simulink model "ArduinoMain"  (R2013a)
settings: Solver=ode3  SolverMode=SingleTasking  StartTime=0.0  StopTime=inf  RelTol=1e-3
PreLoadFcn:
  | load sensorbus
model workspace (MAT data in the model file):
  hc = 23
  zc = -18
  lc = -59
  hsl = -5
  lsl = -28
  rc = 82
undefined symbols (not defined in the file or in its folder): magnitude, sigbuilder_block
libraries: arduinolib x43, simulink x21
settings Model: SimulationMode=external  ExtModeTrigDuration=2  Creator=sbiagion  LastModifiedBy=user
settings OptimizationCC: OptimizeModelRefInitCode=on  LifeSpan=1
settings DebuggingCC: SolverPrmCheckMsg=none  StrictBusMsg=Warning  SFUnusedDataAndEventsDiag=none
settings HardwareCC: ProdBitPerInt=16  ProdBitPerPointer=8  ProdIntDivRoundTo=Zero  ProdEndianess=LittleEndian  ProdWordSize=8  ProdHWDeviceType=Atmel->AVR
settings RTWCC: SystemTargetFile=realtime.tlc  GenerateMakefile=off  TemplateMakefile=realtime.tmf  Description=Run on Target Hardware  RTWVerbose=off  ProcessScript=realtime_make_rtw_hook
settings STFCustomTargetCC: TargetLibSuffix=.a  GenerateSampleERTMain=on  ERTCustomFileBanners=on  SupportNonInlinedSFcns=off  SupportVariableSizeSignals=on  MATLABClassNameForMDSCustomization=Simulink.SoftwareTarget.ERTCustomization  SystemTargetFile=realtime.tlc
settings ERTTargetCC: ParMdlRefBuildCompliant=off  CompOptLevelCompliant=off  ConcurrentExecutionCompliant=off  CombineOutputUpdateFcns=off  ERTFirstTimeCompliant=off  SupportContinuousTime=on  SupportVariableSizeSignals=on  ModelStepFunctionPrototypeControlCompliant=off  CPPClassGenCompliant=off  ExtModeTransport=3  ExtModeMexFile=ext_serial_win32_comm  ExtModeMexArgs=0 15 115200  ERTSrcFileBannerTemplate=realtime_code_template.cgt  ERTHdrFileBannerTemplate=realtime_code_template.cgt  ERTDataSrcFileTemplate=realtime_code_template.cgt  ERTDataHdrFileTemplate=realtime_code_template.cgt  ERTCustomFileTemplate=realtime_file_process.tlc

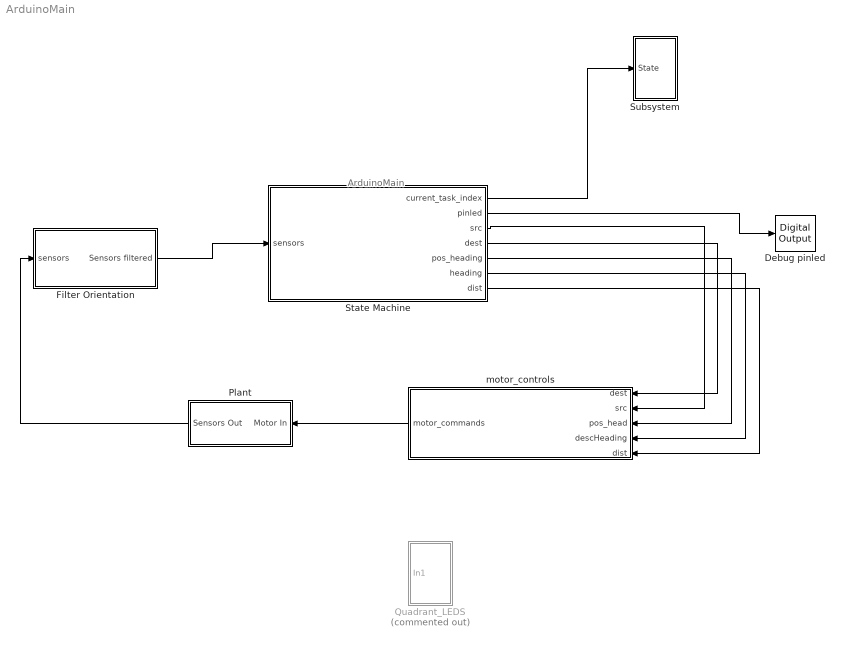
== system ArduinoMain ==
  note: ArduinoMain
  Debug pinled : arduinolib/Digital Output  pinNumber=13
  Filter Orientation : Subsystem
  Plant : Subsystem
  Quadrant_LEDS : Subsystem  Commented=on
  State Machine : Stateflow chart  TreatAsAtomicUnit=on
  Subsystem : Subsystem
  "motor_controls " : Subsystem
  wires:
  State Machine/2(pinled) -> Debug pinled/1
  Plant/1(Sensors Out) -> Filter Orientation/1(sensors)
  Filter Orientation/1(Sensors filtered) -> State Machine/1(sensors)
  "motor_controls "/1("motor_commands ") -> Plant/1(Motor In)
  State Machine/3(src) -> "motor_controls "/2("src ")
  State Machine/4(dest) -> "motor_controls "/1("dest ")
  State Machine/5(pos_heading) -> "motor_controls "/3(pos_head)
  State Machine/6(heading) -> "motor_controls "/4("descHeading ")
  State Machine/7(dist) -> "motor_controls "/5(dist)
  State Machine/1(current_task_index) -> Subsystem/1("State ")

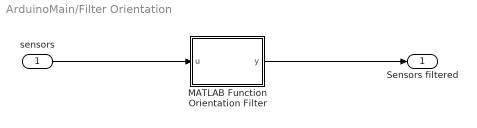
== system ArduinoMain/Filter Orientation ==
  sensors : Inport
  MATLAB Function Orientation Filter : MATLAB Function  TreatAsAtomicUnit=on
  Sensors filtered : Outport
  wires:
  sensors/1 -> MATLAB Function Orientation Filter/1(u)
  MATLAB Function Orientation Filter/1(y) -> Sensors filtered/1

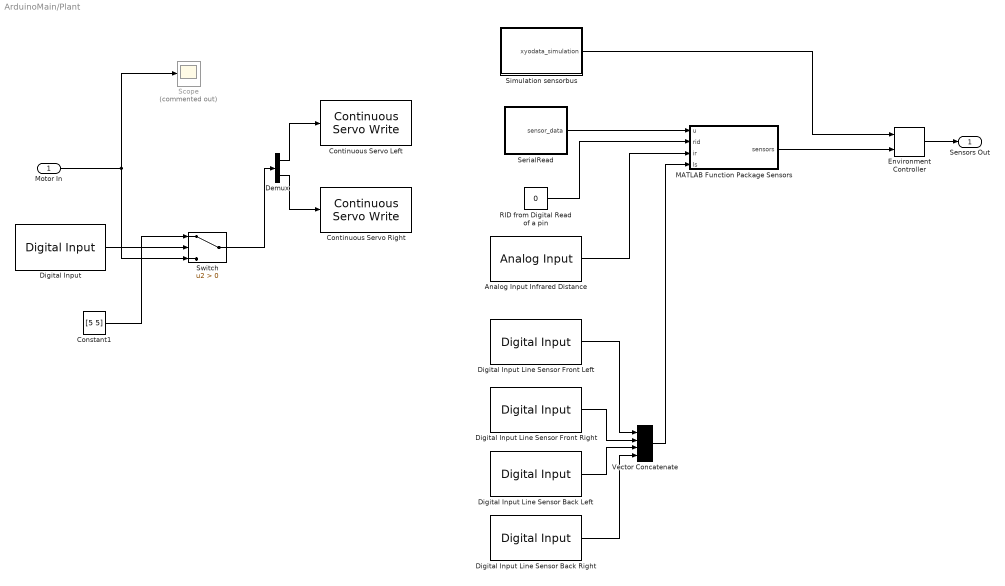
== system ArduinoMain/Plant ==
  Motor In : Inport
  Analog Input Infrared Distance : arduinolib/Analog Input  pinNumber=0  sampleTime=0.01
  Constant1 : Constant  Value=[5 5]
  Continuous Servo Left : arduinolib/Continuous Servo Write  pinNumber=50
  Continuous Servo Right : arduinolib/Continuous Servo Write  pinNumber=51
  Demux : Demux  Outputs=2
  Digital Input : arduinolib/Digital Input  pinNumber=8  sampleTime=1
  Digital Input Line Sensor Back Left : arduinolib/Digital Input  pinNumber=10  sampleTime=0.001
  Digital Input Line Sensor Back Right : arduinolib/Digital Input  pinNumber=11  sampleTime=0.001
  Digital Input Line Sensor Front Left : arduinolib/Digital Input  pinNumber=20  sampleTime=0.001
  Digital Input Line Sensor Front Right : arduinolib/Digital Input  pinNumber=9  sampleTime=0.001
  Environment Controller : simulink/Signal Routing/Environment Controller
  MATLAB Function Package Sensors : MATLAB Function  TreatAsAtomicUnit=on
  RID from Digital Read of a pin : Constant  Value=0  OutDataTypeStr=single  SampleTime=0.001
  Scope : Scope  Commented=on
      settings: ShowLegends=on  YMin=0  YMax=90
  SerialRead : Subsystem
  Simulation sensorbus : Subsystem
  Switch : Switch  Criteria=u2 > Threshold
  Vector Concatenate : Concatenate  NumInputs=4  Mode=Multidimensional array  ConcatenateDimension=2
  Sensors Out : Outport
  wires:
  Demux/2 -> Continuous Servo Right/1
  Demux/1 -> Continuous Servo Left/1
  Motor In/1 -> Scope/1, Switch/3
  Environment Controller/1 -> Sensors Out/1
  Simulation sensorbus/1(xyodata_simulation) -> Environment Controller/1
  Digital Input Line Sensor Front Left/1 -> Vector Concatenate/1
  Digital Input Line Sensor Front Right/1 -> Vector Concatenate/2
  Digital Input Line Sensor Back Left/1 -> Vector Concatenate/3
  Digital Input Line Sensor Back Right/1 -> Vector Concatenate/4
  RID from Digital Read of a pin/1 -> MATLAB Function Package Sensors/2(rid)
  Analog Input Infrared Distance/1 -> MATLAB Function Package Sensors/3(ir)
  Vector Concatenate/1 -> MATLAB Function Package Sensors/4(ls)
  MATLAB Function Package Sensors/1(sensors) -> Environment Controller/2
  SerialRead/1(sensor_data) -> MATLAB Function Package Sensors/1(u)
  Switch/1 -> Demux/1
  Digital Input/1 -> Switch/2
  Constant1/1 -> Switch/1

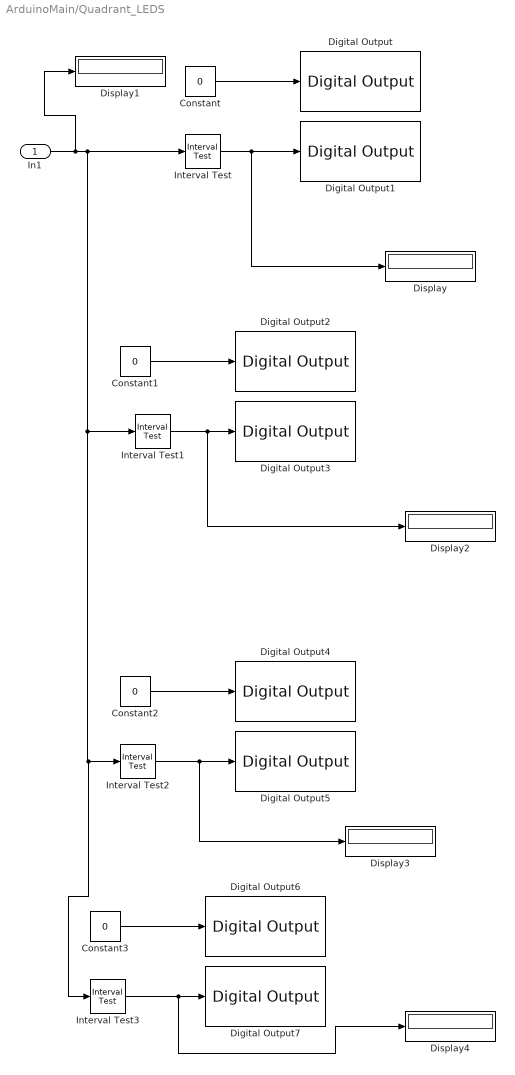
== system ArduinoMain/Quadrant_LEDS ==
  In1 : Inport
  Constant{,1..3} (4 alike) : Constant  Value=0
  Digital Output : arduinolib/Digital Output  pinNumber=23
  Digital Output1 : arduinolib/Digital Output  pinNumber=22
  Digital Output2 : arduinolib/Digital Output  pinNumber=25
  Digital Output3 : arduinolib/Digital Output  pinNumber=24
  Digital Output4 : arduinolib/Digital Output  pinNumber=31
  Digital Output5 : arduinolib/Digital Output  pinNumber=30
  Digital Output6 : arduinolib/Digital Output  pinNumber=29
  Digital Output7 : arduinolib/Digital Output  pinNumber=28
  Display{,1..4} (5 alike) : Display
  Interval Test : simulink/Logic and Bit Operations/Interval Test  IntervalClosedRight=off  uplimit=90  IntervalClosedLeft=on  lowlimit=0  OutDataTypeStr=boolean
  Interval Test1 : simulink/Logic and Bit Operations/Interval Test  IntervalClosedRight=on  uplimit=180  IntervalClosedLeft=on  lowlimit=90  OutDataTypeStr=boolean
  Interval Test2 : simulink/Logic and Bit Operations/Interval Test  IntervalClosedRight=off  uplimit=0  IntervalClosedLeft=on  lowlimit=-90  OutDataTypeStr=boolean
  Interval Test3 : simulink/Logic and Bit Operations/Interval Test  IntervalClosedRight=on  uplimit=-90  IntervalClosedLeft=on  lowlimit=-180  OutDataTypeStr=boolean
  wires:
  Constant/1 -> Digital Output/1
  Interval Test1/1 -> Display2/1, Digital Output3/1
  Constant1/1 -> Digital Output2/1
  Interval Test2/1 -> Display3/1, Digital Output5/1
  Constant2/1 -> Digital Output4/1
  Interval Test/1 -> Display/1, Digital Output1/1
  Interval Test3/1 -> Display4/1, Digital Output7/1
  Constant3/1 -> Digital Output6/1
  In1/1 -> Display1/1, Interval Test/1, Interval Test3/1, Interval Test2/1, Interval Test1/1

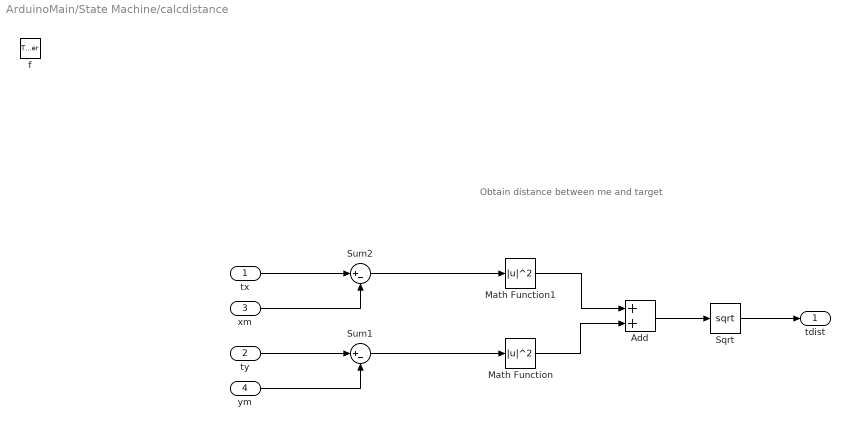
== system ArduinoMain/State Machine/calcdistance ==
  note: Obtain distance between me and target
  tx : Inport  OutDataTypeStr=single  PortDimensions=1
  ty : Inport  Port=2  OutDataTypeStr=single  PortDimensions=1
  xm : Inport  Port=3  OutDataTypeStr=single  PortDimensions=1
  ym : Inport  Port=4  OutDataTypeStr=single  PortDimensions=1
  f : TriggerPort  TriggerType=function-call
      settings: CopyFcn=Stateflow.SLINSF.SimulinkMan.removeBlockPreDeleteFcn  PreDeleteFcn=Stateflow.SLINSF.SimulinkMan.unsafePredeleteFcn
  Add : Sum
  Math Function : Math  Operator=magnitude^2  SaturateOnIntegerOverflow=on
  Math Function1 : Math  Operator=magnitude^2  SaturateOnIntegerOverflow=on
  Sqrt : Sqrt  SaturateOnIntegerOverflow=on
  Sum1 : Sum  Inputs=|+-
  Sum2 : Sum  Inputs=|+-
  tdist : Outport
  wires:
  ty/1 -> Sum1/1
  ym/1 -> Sum1/2
  tx/1 -> Sum2/1
  xm/1 -> Sum2/2
  Sum1/1 -> Math Function/1
  Sum2/1 -> Math Function1/1
  Add/1 -> Sqrt/1
  Math Function1/1 -> Add/1
  Math Function/1 -> Add/2
  Sqrt/1 -> tdist/1

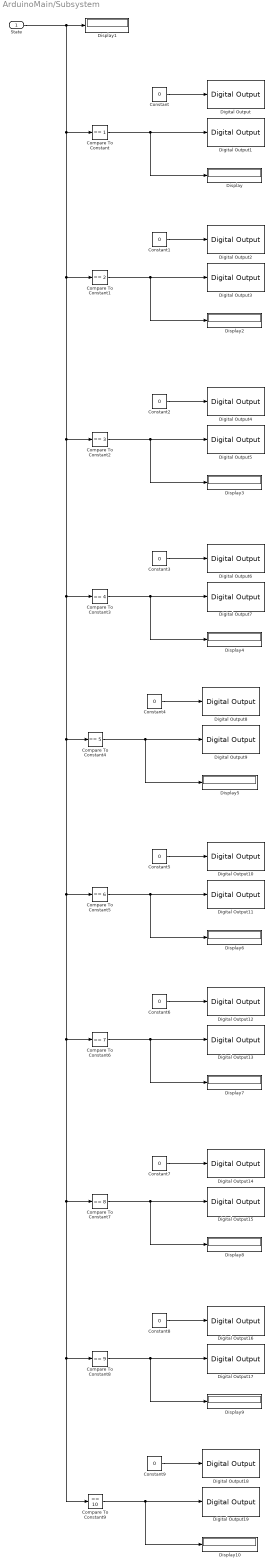
== system ArduinoMain/Subsystem ==
  "State " : Inport
  Compare To Constant : simulink/Logic and Bit Operations/Compare To Constant  relop===  const=1  OutDataTypeStr=boolean
  Compare To Constant1 : simulink/Logic and Bit Operations/Compare To Constant  relop===  const=2  OutDataTypeStr=boolean
  Compare To Constant2 : simulink/Logic and Bit Operations/Compare To Constant  relop===  const=3  OutDataTypeStr=boolean
  Compare To Constant3 : simulink/Logic and Bit Operations/Compare To Constant  relop===  const=4  OutDataTypeStr=boolean
  Compare To Constant4 : simulink/Logic and Bit Operations/Compare To Constant  relop===  const=5  OutDataTypeStr=boolean
  Compare To Constant5 : simulink/Logic and Bit Operations/Compare To Constant  relop===  const=6  OutDataTypeStr=boolean
  Compare To Constant6 : simulink/Logic and Bit Operations/Compare To Constant  relop===  const=7  OutDataTypeStr=boolean
  Compare To Constant7 : simulink/Logic and Bit Operations/Compare To Constant  relop===  const=8  OutDataTypeStr=boolean
  Compare To Constant8 : simulink/Logic and Bit Operations/Compare To Constant  relop===  const=9  OutDataTypeStr=boolean
  Compare To Constant9 : simulink/Logic and Bit Operations/Compare To Constant  relop===  const=10  OutDataTypeStr=boolean
  Constant{,1..9} (10 alike) : Constant  Value=0
  Digital Output : arduinolib/Digital Output  pinNumber=23
  Digital Output1 : arduinolib/Digital Output  pinNumber=22
  Digital Output10 : arduinolib/Digital Output  pinNumber=33
  Digital Output11 : arduinolib/Digital Output  pinNumber=32
  Digital Output12 : arduinolib/Digital Output  pinNumber=35
  Digital Output13 : arduinolib/Digital Output  pinNumber=34
  Digital Output14 : arduinolib/Digital Output  pinNumber=37
  Digital Output15 : arduinolib/Digital Output  pinNumber=36
  Digital Output16 : arduinolib/Digital Output  pinNumber=39
  Digital Output17 : arduinolib/Digital Output  pinNumber=38
  Digital Output18 : arduinolib/Digital Output  pinNumber=41
  Digital Output19 : arduinolib/Digital Output  pinNumber=40
  Digital Output2 : arduinolib/Digital Output  pinNumber=25
  Digital Output3 : arduinolib/Digital Output  pinNumber=24
  Digital Output4 : arduinolib/Digital Output  pinNumber=27
  Digital Output5 : arduinolib/Digital Output  pinNumber=26
  Digital Output6 : arduinolib/Digital Output  pinNumber=29
  Digital Output7 : arduinolib/Digital Output  pinNumber=28
  Digital Output8 : arduinolib/Digital Output  pinNumber=31
  Digital Output9 : arduinolib/Digital Output  pinNumber=30
  Display{,1..10} (11 alike) : Display
  wires:
  Constant/1 -> Digital Output/1
  Compare To Constant/1 -> Display/1, Digital Output1/1
  Constant1/1 -> Digital Output2/1
  Compare To Constant1/1 -> Display2/1, Digital Output3/1
  Constant2/1 -> Digital Output4/1
  Compare To Constant2/1 -> Display3/1, Digital Output5/1
  Constant3/1 -> Digital Output6/1
  Compare To Constant3/1 -> Display4/1, Digital Output7/1
  Constant4/1 -> Digital Output8/1
  Compare To Constant4/1 -> Display5/1, Digital Output9/1
  Constant5/1 -> Digital Output10/1
  Compare To Constant5/1 -> Display6/1, Digital Output11/1
  Constant6/1 -> Digital Output12/1
  Compare To Constant6/1 -> Display7/1, Digital Output13/1
  Constant7/1 -> Digital Output14/1
  Compare To Constant7/1 -> Display8/1, Digital Output15/1
  "State "/1 -> Compare To Constant9/1, Compare To Constant8/1, Compare To Constant7/1, Compare To Constant6/1, Compare To Constant5/1, Compare To Constant4/1, Compare To Constant3/1, Compare To Constant2/1, Compare To Constant1/1, Compare To Constant/1, Display1/1
  Constant8/1 -> Digital Output16/1
  Compare To Constant8/1 -> Display9/1, Digital Output17/1
  Constant9/1 -> Digital Output18/1
  Compare To Constant9/1 -> Display10/1, Digital Output19/1

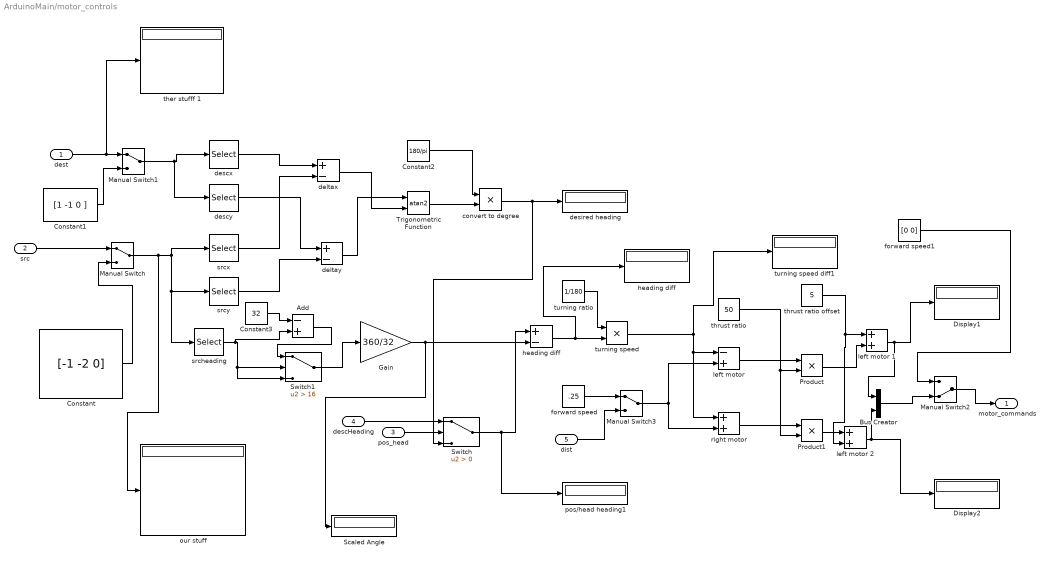
== system ArduinoMain/motor_controls  ==
  "dest " : Inport
  "src " : Inport  Port=2
  pos_head : Inport  Port=3  OutDataTypeStr=boolean
  "descHeading " : Inport  Port=4
  dist : Inport  Port=5
  Add : Sum  Inputs=-+
  Bus Creator : BusCreator  Inputs=2
  Constant : Constant  Value=[-1 -2 0]
  Constant1 : Constant  Value=[1 -1 0 ]
  Constant2 : Constant  Value=180/pi
  Constant3 : Constant  Value=32
  Display1 : Display
  Display2 : Display
  Gain : Gain  Gain=360/32
  Manual Switch : ManualSwitch
  Manual Switch1 : ManualSwitch
  Manual Switch2 : ManualSwitch  CurrentSetting=0
  Manual Switch3 : ManualSwitch
  Product : Product
  Product1 : Product
  Scaled Angle : Display
  Switch : Switch  Criteria=u2 > Threshold
  Switch1 : Switch  Criteria=u2 > Threshold  Threshold=16
  Trigonometric Function : Trigonometry  Operator=atan2
  "convert to degree " : Product
  deltax : Sum  Inputs=+-
  deltay : Sum  Inputs=+-
  "descx " : Selector  InputPortWidth=3  IndexOptions=Index vector (dialog)  Indices=1  OutputSizes=1
  "descy " : Selector  InputPortWidth=3  IndexOptions=Index vector (dialog)  Indices=2  OutputSizes=1
  "desired heading " : Display
  forward speed : Constant  Value=.25
  forward speed1 : Constant  Value=[0 0]
  heading diff : Display
  "heading diff " : Sum  Inputs=+-
  "left motor " : Sum  Inputs=-+
  left motor 1 : Sum
  left motor 2 : Sum
  "our stuff " : Display
  pos/head heading1 : Display
  "right motor " : Sum
  "srcheading " : Selector  InputPortWidth=3  IndexOptions=Index vector (dialog)  Indices=3  OutputSizes=1
  "srcx " : Selector  InputPortWidth=3  IndexOptions=Index vector (dialog)  Indices=1  OutputSizes=1
  "srcy " : Selector  InputPortWidth=3  IndexOptions=Index vector (dialog)  Indices=2  OutputSizes=1
  ther stufff 1 : Display
  "thrust ratio " : Constant  Value=50
  thrust ratio offset : Constant  Value=5
  turning ratio : Constant  Value=1/180
  turning speed : Product
  turning speed diff1 : Display
  "motor_commands " : Outport
  wires:
  "descx "/1 -> deltax/1
  "srcx "/1 -> deltax/2
  "descy "/1 -> deltay/1
  "srcy "/1 -> deltay/2
  deltax/1 -> Trigonometric Function/2
  deltay/1 -> Trigonometric Function/1
  Trigonometric Function/1 -> "convert to degree "/2
  "convert to degree "/1 -> Switch/3, "desired heading "/1
  Constant2/1 -> "convert to degree "/1
  "heading diff "/1 -> turning speed/2, heading diff/1
  turning ratio/1 -> turning speed/1
  turning speed/1 -> turning speed diff1/1, "right motor "/1, "left motor "/1
  "left motor "/1 -> Product/1
  "right motor "/1 -> Product1/1
  "thrust ratio "/1 -> Product1/2, Product/2
  pos_head/1 -> Switch/2
  Switch/1 -> pos/head heading1/1, "heading diff "/1
  Product/1 -> left motor 1/2
  left motor 1/1 -> Bus Creator/1, Display1/1
  thrust ratio offset/1 -> left motor 2/2, left motor 1/1
  Product1/1 -> left motor 2/1
  left motor 2/1 -> Display2/1, Bus Creator/2
  "dest "/1 -> ther stufff 1/1, Manual Switch1/1
  Manual Switch1/1 -> "descy "/1, "descx "/1
  "src "/1 -> Manual Switch/1
  Manual Switch/1 -> "our stuff "/1, "srcx "/1, "srcheading "/1, "srcy "/1
  Constant/1 -> Manual Switch/2
  Constant1/1 -> Manual Switch1/2
  Bus Creator/1 -> Manual Switch2/2
  Manual Switch2/1 -> "motor_commands "/1
  forward speed1/1 -> Manual Switch2/1
  "descHeading "/1 -> Switch/1
  forward speed/1 -> Manual Switch3/1
  Manual Switch3/1 -> "left motor "/2, "right motor "/2
  dist/1 -> Manual Switch3/2
  "srcheading "/1 -> Add/2, Switch1/3, Switch1/2
  Switch1/1 -> Gain/1
  Add/1 -> Switch1/1
  Constant3/1 -> Add/1
  Gain/1 -> Scaled Angle/1, "heading diff "/2

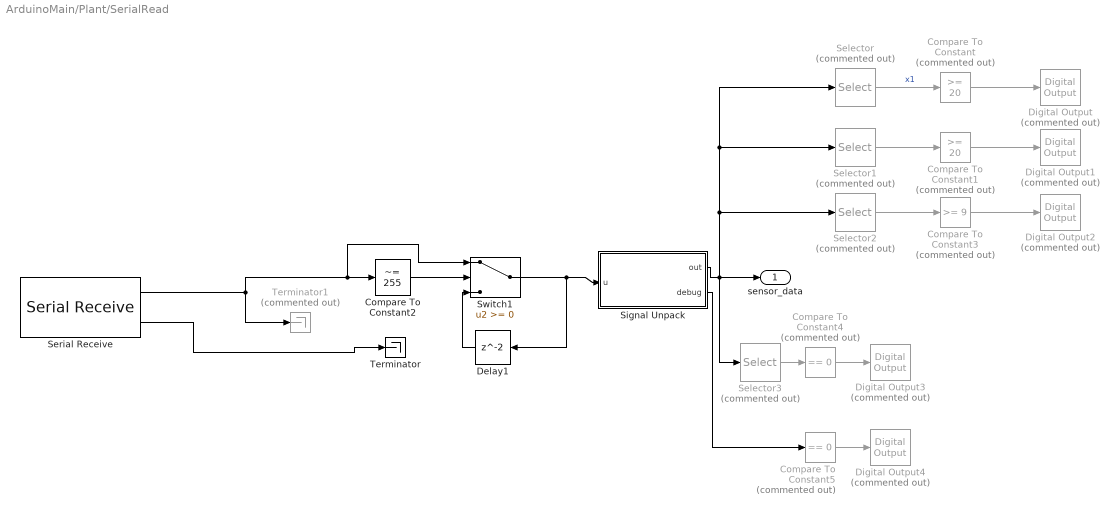
== system ArduinoMain/Plant/SerialRead ==
  Compare To Constant : simulink/Logic and Bit Operations/Compare To Constant  Commented=on  relop=>=  const=20  OutDataTypeStr=boolean
  Compare To Constant1 : simulink/Logic and Bit Operations/Compare To Constant  Commented=on  relop=>=  const=20  OutDataTypeStr=boolean
  Compare To Constant2 : simulink/Logic and Bit Operations/Compare To Constant  relop=~=  const=255  OutDataTypeStr=boolean
  Compare To Constant3 : simulink/Logic and Bit Operations/Compare To Constant  Commented=on  relop=>=  const=9  OutDataTypeStr=boolean
  Compare To Constant4 : simulink/Logic and Bit Operations/Compare To Constant  Commented=on  relop===  const=0  OutDataTypeStr=boolean
  Compare To Constant5 : simulink/Logic and Bit Operations/Compare To Constant  Commented=on  relop===  const=0  OutDataTypeStr=boolean
  Delay1 : Delay
  Digital Output : arduinolib/Digital Output  Commented=on  pinNumber=12
  Digital Output1 : arduinolib/Digital Output  Commented=on  pinNumber=11
  Digital Output2 : arduinolib/Digital Output  Commented=on  pinNumber=10
  Digital Output3 : arduinolib/Digital Output  Commented=on  pinNumber=9
  Digital Output4 : arduinolib/Digital Output  Commented=on  pinNumber=9
  Selector : Selector  Commented=on  InputPortWidth=7  IndexOptions=Index vector (dialog)  Indices=1  OutputSizes=1
  Selector1 : Selector  Commented=on  InputPortWidth=7  IndexOptions=Index vector (dialog)  Indices=2  OutputSizes=1
  Selector2 : Selector  Commented=on  InputPortWidth=7  IndexOptions=Index vector (dialog)  Indices=3  OutputSizes=1
  Selector3 : Selector  Commented=on  InputPortWidth=7  IndexOptions=Index vector (dialog)  Indices=7  OutputSizes=1
  Serial Receive : arduinolib/Serial Receive  portNumber=1  showOutStatus=on  sampleTime=0.001
  Signal Unpack : MATLAB Function  TreatAsAtomicUnit=on
  Switch1 : Switch
  Terminator : Terminator
  Terminator1 : Terminator  Commented=on
  sensor_data : Outport
  wires:
  Switch1/1 -> Delay1/1, Signal Unpack/1(u)
  Compare To Constant2/1 -> Switch1/2
  Serial Receive/2 -> Terminator/1
  Delay1/1 -> Switch1/3
  Serial Receive/1 -> Terminator1/1, Switch1/1, Compare To Constant2/1
  Selector/1 -> Compare To Constant/1  "x1"
  Compare To Constant/1 -> Digital Output/1
  Compare To Constant1/1 -> Digital Output1/1
  Selector1/1 -> Compare To Constant1/1
  Selector2/1 -> Compare To Constant3/1
  Compare To Constant3/1 -> Digital Output2/1
  Selector3/1 -> Compare To Constant4/1
  Signal Unpack/1(out) -> Selector3/1, Selector/1, Selector1/1, Selector2/1, sensor_data/1
  Compare To Constant4/1 -> Digital Output3/1
  Signal Unpack/2(debug) -> Compare To Constant5/1
  Compare To Constant5/1 -> Digital Output4/1

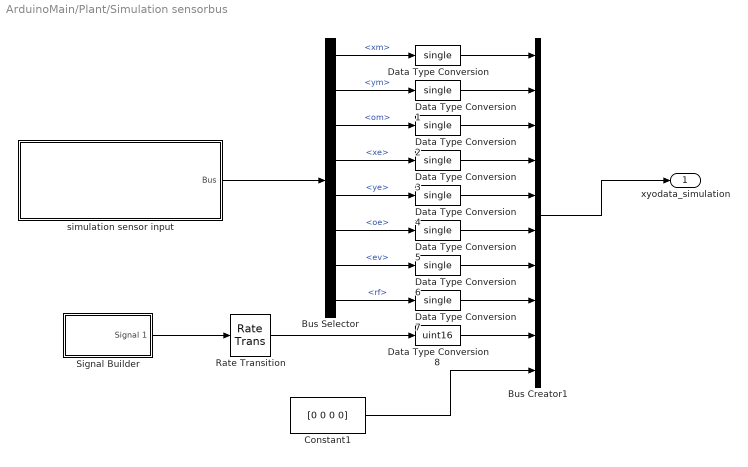
== system ArduinoMain/Plant/Simulation sensorbus ==
  Bus Creator1 : BusCreator  Inputs=10  OutDataTypeStr=Bus: sensorbus  NonVirtualBus=on
  Bus Selector : BusSelector  OutputSignals=xm,ym,om,xe,ye,oe,ev,rf
  Constant1 : Constant  Value=[0 0 0 0]  OutDataTypeStr=boolean
  Data Type Conversion{,1..7} (8 alike) : DataTypeConversion  OutDataTypeStr=single
  Data Type Conversion8 : DataTypeConversion  OutDataTypeStr=uint16
  Rate Transition : RateTransition  Integrity=off
  Signal Builder : Subsystem  Tag=STV Subsys  LoadFcn=sigbuilder_block('load');  StartFcn=sigbuilder_block('start');  StopFcn=sigbuilder_block('stop');  ClipboardFcn=sigbuilder_block('clipboard');  mask(Sigbuilder block){}
      mask help: Simulink:masks:SigbuilderBlock_MD
      mask init:
      | if ~strcmp(get_param(bdroot(gcbh),'SimulationStatus'),'stopped') tuvar = sigbuilder_block('maskInit'); end
      settings: CopyFcn=sigbuilder_block('copy');  DeleteFcn=sigbuilder_block('delete');  ModelCloseFcn=sigbuilder_block('modelClose');  PreSaveFcn=sigbuilder_block('preSave');  PauseFcn=sigbuilder_block('pause');  ContinueFcn=sigbuilder_block('continue');  NameChangeFcn=sigbuilder_block('namechange');  OpenFcn=sigbuilder_block('open',[437.25 199.5 550.5 399.75 ]);  CloseFcn=sigbuilder_block('close');
      mask Display: plot(0, 0, 100, 100,[2, 2, 32, 32, 2], [68, 8, 8, 68, 68],[32, 2], [38, 38], [32, 19, 2],[53, 60, 44], [32, 17, 17, 2],[16, 16, 31, 31]);txt = getActiveGroup(gcbh);text(2, 100, txt,'verticalAlignment', 'top');
  simulation sensor input : Subsystem  Tag=STV Subsys  LoadFcn=sigbuilder_block('load');  StartFcn=sigbuilder_block('start');  StopFcn=sigbuilder_block('stop');  ClipboardFcn=sigbuilder_block('clipboard');  mask(Sigbuilder block){}
      mask help: Simulink:masks:SigbuilderBlock_MD
      mask init:
      | if ~strcmp(get_param(bdroot(gcbh),'SimulationStatus'),'stopped') tuvar = sigbuilder_block('maskInit'); end
      settings: CopyFcn=sigbuilder_block('copy');  DeleteFcn=sigbuilder_block('delete');  ModelCloseFcn=sigbuilder_block('modelClose');  PreSaveFcn=sigbuilder_block('preSave');  PauseFcn=sigbuilder_block('pause');  ContinueFcn=sigbuilder_block('continue');  NameChangeFcn=sigbuilder_block('namechange');  OpenFcn=sigbuilder_block('open',[6 21 948 684 ]);  CloseFcn=sigbuilder_block('close');
      mask Display: plot(0, 0, 100, 100,[2, 2, 32, 32, 2], [68, 8, 8, 68, 68],[32, 2], [38, 38], [32, 19, 2],[53, 60, 44], [32, 17, 17, 2],[16, 16, 31, 31]);txt = getActiveGroup(gcbh);text(2, 100, txt,'verticalAlignment', 'top');
  xyodata_simulation : Outport  OutDataTypeStr=Bus: sensorbus
  wires:
  simulation sensor input/1(Bus) -> Bus Selector/1
  Bus Selector/1 -> Data Type Conversion/1  "<xm>"
  Bus Creator1/1 -> xyodata_simulation/1
  Bus Selector/3 -> Data Type Conversion2/1  "<om>"
  Bus Selector/2 -> Data Type Conversion1/1  "<ym>"
  Bus Selector/5 -> Data Type Conversion4/1  "<ye>"
  Bus Selector/6 -> Data Type Conversion5/1  "<oe>"
  Bus Selector/7 -> Data Type Conversion6/1  "<ev>"
  Bus Selector/8 -> Data Type Conversion7/1  "<rf>"
  Bus Selector/4 -> Data Type Conversion3/1  "<xe>"
  Data Type Conversion/1 -> Bus Creator1/1
  Data Type Conversion1/1 -> Bus Creator1/2
  Data Type Conversion2/1 -> Bus Creator1/3
  Data Type Conversion3/1 -> Bus Creator1/4
  Data Type Conversion4/1 -> Bus Creator1/5
  Data Type Conversion5/1 -> Bus Creator1/6
  Data Type Conversion6/1 -> Bus Creator1/7
  Data Type Conversion7/1 -> Bus Creator1/8
  Signal Builder/1(Signal 1) -> Rate Transition/1
  Constant1/1 -> Bus Creator1/10
  Data Type Conversion8/1 -> Bus Creator1/9
  Rate Transition/1 -> Data Type Conversion8/1

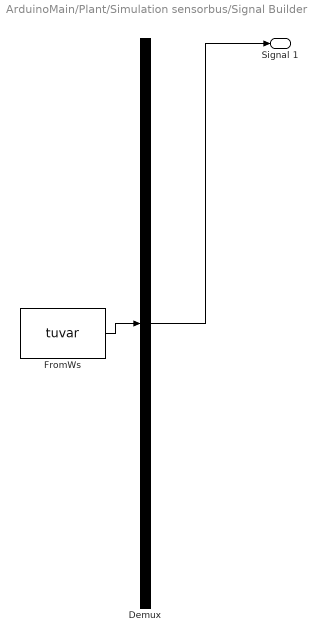
== system ArduinoMain/Plant/Simulation sensorbus/Signal Builder ==
  Demux : Demux  Tag=STV Demux  Outputs=1
  FromWs : FromWorkspace  Tag=STV FromWs  VariableName=tuvar  SampleTime=0.01
      SigBuilderData=|
      | common.afterFinalStr = 'Extrapolate'
      | common.sampleTime = '0.01'
      | dataSet.timeRange = [0 10]
      | dataSet.name = 'Group 1'
      | sbobj.Groups.Name = 'Group 1'
      | sbobj.Groups.Signals.Name = 'Signal 1'
      | sbobj.Groups.Signals.XData = [0 1 1 2 2 3 10]
      | sbobj.Groups.Signals.YData = [0 0 100 100 200 200 200]
  Signal 1 : Outport  Tag=STV Outport
  wires:
  Demux/1 -> Signal 1/1
  FromWs/1 -> Demux/1

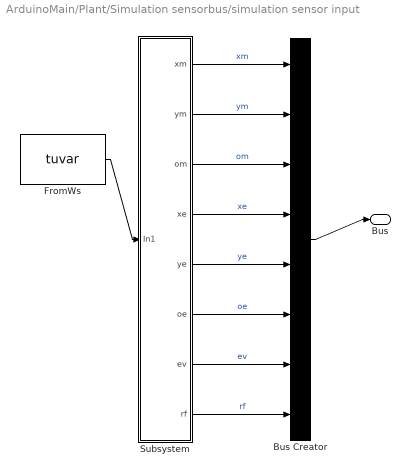
== system ArduinoMain/Plant/Simulation sensorbus/simulation sensor input ==
  Bus Creator : BusCreator  Tag=Bus Creator  Inputs=8
  FromWs : FromWorkspace  Tag=STV FromWs  VariableName=tuvar  SampleTime=0.001  OutputAfterFinalValue=Holding final value
      SigBuilderData=|
      | common.afterFinalStr = 'Hold final value'
      | common.sampleTime = '0.001'
      | dataSet(1).timeRange = [0 18]
      | dataSet(1).name = 'Navigate to a point and return to original'
      | dataSet(2).timeRange = [0 18]
      | dataSet(2).name = 'Navigate from center to edge'
      | sbobj.Groups(1).Name = 'Navigate to a point and return to original'
      | sbobj.Groups(1).Signals(1).Name = 'xm'
      | sbobj.Groups(1).Signals(1).XData = [0 6 8 14 18]
      | sbobj.Groups(1).Signals(1).YData = [24 0 0 24 24]
      | sbobj.Groups(1).Signals(2).Name = 'ym'
      | sbobj.Groups(1).Signals(2).XData = [0 6 8 14 18]
      | sbobj.Groups(1).Signals(2).YData = [10 23 23 10 10]
      | sbobj.Groups(1).Signals(3).Name = 'om'
      | sbobj.Groups(1).Signals(3).XData = [0 6 8 18]
      | sbobj.Groups(1).Signals(3).YData = [12 12 24 24]
      | sbobj.Groups(1).Signals(4).Name = 'xe'
      | sbobj.Groups(1).Signals(4).XData = [0 18]
      | sbobj.Groups(1).Signals(4).YData = [24 24]
      | sbobj.Groups(1).Signals(5).Name = 'ye'
      | sbobj.Groups(1).Signals(5).XData = [0 18]
      | sbobj.Groups(1).Signals(5).YData = [10 10]
      | sbobj.Groups(1).Signals(6).Name = 'oe'
      | sbobj.Groups(1).Signals(6).XData = [0 18]
      | sbobj.Groups(1).Signals(6).YData = [0 0]
      | sbobj.Groups(1).Signals(7).Name = 'ev'
      | sbobj.Groups(1).Signals(7).XData = [0 18]
      | sbobj.Groups(1).Signals(7).YData = [0 0]
      | sbobj.Groups(1).Signals(8).Name = 'rf'
      | sbobj.Groups(1).Signals(8).XData = [0 18]
      | sbobj.Groups(1).Signals(8).YData = [1 1]
      | sbobj.Groups(1).TimeRange = [0 18]
      | sbobj.Groups(2).Name = 'Navigate from center to edge'
      | sbobj.Groups(2).Signals(1).Name = 'xm'
      | sbobj.Groups(2).Signals(1).XData = [0 10 18]
      | sbobj.Groups(2).Signals(1).YData = [1 32 32]
      | sbobj.Groups(2).Signals(2).Name = 'ym'
      | sbobj.Groups(2).Signals(2).XData = [0 18]
      | sbobj.Groups(2).Signals(2).YData = [16 16]
      | sbobj.Groups(2).Signals(3).Name = 'om'
      | sbobj.Groups(2).Signals(3).XData = [0 18]
      | sbobj.Groups(2).Signals(3).YData = [0 0]
      | sbobj.Groups(2).Signals(4).Name = 'xe'
      | sbobj.Groups(2).Signals(4).XData = [0 18]
      | sbobj.Groups(2).Signals(4).YData = [24 24]
      | sbobj.Groups(2).Signals(5).Name = 'ye'
      | sbobj.Groups(2).Signals(5).XData = [0 18]
      | sbobj.Groups(2).Signals(5).YData = [10 10]
      | sbobj.Groups(2).Signals(6).Name = 'oe'
      | sbobj.Groups(2).Signals(6).XData = [0 18]
      | sbobj.Groups(2).Signals(6).YData = [0 0]
      | sbobj.Groups(2).Signals(7).Name = 'ev'
      | sbobj.Groups(2).Signals(7).XData = [0 18]
      | sbobj.Groups(2).Signals(7).YData = [0 0]
      | sbobj.Groups(2).Signals(8).Name = 'rf'
      | sbobj.Groups(2).Signals(8).XData = [0 18]
      | sbobj.Groups(2).Signals(8).YData = [1 1]
      | sbobj.Groups(2).TimeRange = [0 18]
  Subsystem : Subsystem
  Bus : Outport
  wires:
  FromWs/1 -> Subsystem/1(In1)
  Subsystem/1(xm) -> Bus Creator/1  "xm"
  Subsystem/2(ym) -> Bus Creator/2  "ym"
  Bus Creator/1 -> Bus/1
  Subsystem/3(om) -> Bus Creator/3  "om"
  Subsystem/4(xe) -> Bus Creator/4  "xe"
  Subsystem/5(ye) -> Bus Creator/5  "ye"
  Subsystem/6(oe) -> Bus Creator/6  "oe"
  Subsystem/7(ev) -> Bus Creator/7  "ev"
  Subsystem/8(rf) -> Bus Creator/8  "rf"

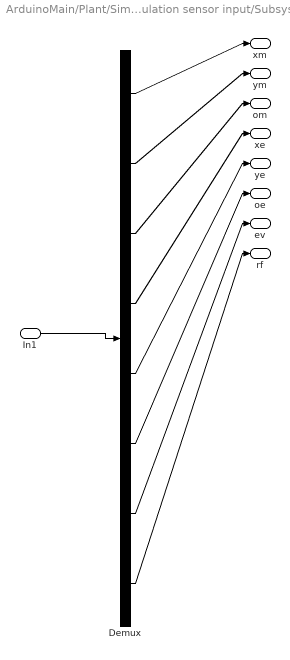
== system ArduinoMain/Plant/Simulation sensorbus/simulation sensor input/Subsystem ==
  In1 : Inport
  Demux : Demux  Tag=STV Demux  Outputs=8
  xm : Outport  Tag=STV Outport
  ym : Outport  Tag=STV Outport  Port=2
  om : Outport  Tag=STV Outport  Port=3
  xe : Outport  Tag=STV Outport  Port=4
  ye : Outport  Tag=STV Outport  Port=5
  oe : Outport  Tag=STV Outport  Port=6
  ev : Outport  Tag=STV Outport  Port=7
  rf : Outport  Tag=STV Outport  Port=8
  wires:
  Demux/1 -> xm/1
  Demux/2 -> ym/1
  In1/1 -> Demux/1
  Demux/3 -> om/1
  Demux/4 -> xe/1
  Demux/5 -> ye/1
  Demux/6 -> oe/1
  Demux/7 -> ev/1
  Demux/8 -> rf/1

== matlab function ArduinoMain/Plant/SerialRead/Signal Unpack ==
  data: u input uint8 size=[1 1]; out output single size=[1 7]; debug output single
function [out, debug] = fcn(u)
%lofunction [out,debug]  = fcn(u)
%#codegen
persistent x1temp x2temp y1temp y2temp o1temp o2temp rftemp debugtemp
if isempty(x1temp)
    x1temp = single(0);
end
if isempty(x2temp)
    x2temp = single(0);
end
if isempty(y1temp)
    y1temp = single(0);
end
if isempty(y2temp)
    y2temp = single(0);
end
if isempty(o1temp)
    o1temp = single(0);
end
if isempty(o2temp)
    o2temp = single(0);
end
if isempty(rftemp)
    rftemp = single(0);
end
if isempty(debugtemp)
    debugtemp = single(0);
end

x1 = single(0); x2 = single(0); y1 = single(0); y2 = single(0); 
o1 = single(0); o2 = single(0); rf = single(0);

% unpack data
inbits = de2bimod(u,8);
id = inbits(1:3);
if isequal(id,[0 0 0])
    % update x data
    x1 = single(bi2demod(inbits(4:8)));
    x2 = x2temp;
    y1 = y1temp;
    y2 = y2temp;
    o1 = o1temp;
    o2 = o2temp;
    rf = rftemp;
    % update old x1 data
    x1temp = x1;
elseif isequal(id,[1 0 0])
    % update y data
    x1 = x1temp;
    x2 = x2temp;
    y1 = single(bi2demod(inbits(4:8)));
    y2 = y2temp;
    o1 = o1temp;
    o2 = o2temp;
    rf = rftemp;
    % update old y1 data
    y1temp = y1;
elseif isequal(id,[0 1 0])
    % update orientation data;
    x1 = x1temp;
    x2 = x2temp;
    y1 = y1temp;
    y2 = y2temp;
    o1 = single(bi2demod(inbits(4:8)));
    o2 = o2temp;
    rf = rftemp;
    % update old o1 data
    o1temp = o1;
elseif isequal(id,[1 1 0])
    x1 = x1temp;
    x2 = single(bi2demod(inbits(4:8)));
    y1 = y1temp;
    y2 = y2temp;
    o1 = o1temp;
    o2 = o2temp;
    rf = rftemp;
    % update old x2 data
    x2temp = x2;
elseif isequal(id,[0 0 1])
    x1 = x1temp;
    x2 = x2temp;
    y1 = y1temp;
    y2 = single(bi2demod(inbits(4:8)));
    o1 = o1temp;
    o2 = o2temp;
    rf = rftemp;
    % update old y2 data
    y2temp = y2;
elseif isequal(id,[1 0 1])
    x1 = x1temp;
    x2 = x2temp;
    y1 = y1temp;
    y2 = y2temp;
    o1 = o1temp;
    o2 = single(bi2demod(inbits(4:8)));
    rf = rftemp;
    % update old o2 data
    o2temp = o2;
elseif isequal(id,[0 1 1])
    x1 = x1temp;
    x2 = x2temp;
    y1 = y1temp;
    y2 = y2temp;
    o1 = o1temp;
    o2 = o2temp;
    rf = single(bi2demod(inbits(4:8)));
    % update persistent rf variable
    rftemp = rf;
    debugtemp = single(1);
end

debug = debugtemp;

out = [x1 y1 o1 x2 y2 o2 rf];

== matlab function ArduinoMain/Plant/MATLAB Function Package Sensors ==
  data: u input single; sensors output Bus: sensorbus; rid input single; ir input; ls input
function sensors = fcn(u,rid,ir,ls)
%#codegen
xm = single(0); ym = single(0); om = single(0); 
xe = single(0); ye = single(0); oe = single(0);
if rid == 0
    xm = u(1);
    ym = u(2);
    om = u(3);
    xe = u(4);
    ye = u(5);
    oe = u(6);
elseif rid == 1
    xm = u(4);
    ym = u(5);
    om = u(6);
    xe = u(1);
    ye = u(2);
    oe = u(3);
end
ev = atan2(ye-ym,xe-xm)*16/pi+16; % 0 to 32
rf = u(7);

% package sensorbus
sensors.xm = xm; % x of me
sensors.ym = ym; % y of me
sensors.om = om; % orientation of me
sensors.xe = xe; % x of enemy
sensors.ye = ye; % y of enemy
sensors.oe = oe; % orientation of enemy
sensors.ev = ev; % enemy vector
sensors.rf = rf; % run flag
sensors.ir = ir; % infrared sensor
sensors.ls = ls; % line sensors [1 4]

== matlab function ArduinoMain/Filter Orientation/MATLAB Function Orientation Filter ==
  data: u input Bus: sensorbus; y output Bus: sensorbus
function y = fcn(u)
%#codegen
persistent o1temp 
if isempty(o1temp)
    o1temp = single(0);
end

if (o1temp - u.om)>=16
    u.om = o1temp;
end
o1temp = u.om;         
y = u;

== stateflow chart ArduinoMain/State Machine ==
  settings: updateMethod=DISCRETE  sampleTime=0.01
  state normal_operation
    during:
    t1 = t1 - 1;
    state current_task
      state task1
        % check run flag
        entry:
        checkrun;
      state task2
        % stop motor due to run flag
        entry:
        stopmotor;
      state task3
        % check distance task
        entry:
        checkdistance;
      state task4
        % main task
        entry:
        maintask;
      state task5
        % navigate to target x-y
        entry:
      state task6
        % perform close maneuvers
        entry:
        closetask;
      state task7
        % debug test motor state
        entry:
        test_motor
      state task8
        % IR track object state
        entry:
        irtrack;
      state task9
        % avoid line
        entry:
        avoidline;
      state task10
        % avoid line
        entry:
        testdrewnotsucking;
      state debug
        entry:
    (default) -> (junction 8) : {current_task_index = single(1);}
    (junction 14) -> (junction 8)
    current_task -> (junction 14)
    (junction 8) -> (junction 22)
    (junction 22) -> task1 [order 1] : [current_task_index == 1 && t1<=0]
    (junction 22) -> (junction 120) [order 2]
    (junction 120) -> task2 [order 1] : [current_task_index == 2 && t1<=0]
    (junction 120) -> (junction 133) [order 2]
    (junction 133) -> task3 [order 1] : [current_task_index == 3 && t1<=0]
    (junction 133) -> (junction 24) [order 2]
    (junction 24) -> task4 [order 1] : [current_task_index == 4 && t1<=0]
    (junction 24) -> (junction 86) [order 2]
    (junction 86) -> task5 [order 1] : [current_task_index == 5 && t1 <=0]
    (junction 86) -> (junction 124) [order 2]
    (junction 124) -> task6 [order 1] : [current_task_index == 6 && t1 <=0]
    (junction 124) -> (junction 113) [order 2]
    (junction 113) -> task7 [order 1] : [current_task_index == 7 && t1<=0]
    (junction 113) -> (junction 152) [order 2]
    (junction 152) -> task8 [order 1] : [current_task_index == 8 && t1<=0]
    (junction 152) -> (junction 158) [order 2]
    (junction 158) -> task9 [order 1] : [current_task_index == 9 && t1<=0]
    (junction 158) -> (junction 182) [order 2]
    (junction 182) -> task10 [order 1] : [current_task_index ==10 && t1<=0]
    (junction 182) -> debug [order 2]
  state tdist = calcdistance(tx,ty,xm,ym) [function]
  (default) -> normal_operation : {initialization;}
  data: tx function_input single size=1; ty function_input single size=1; xm function_input single size=1; ym function_input single size=1; tdist function_output; sensors input Bus: sensorbus; current_task_index output single; debug_normal local boolean; enter_flag local boolean; t1 local single size=1; t2 local single size=1; t3 local single size=1; ty local single; tx local single; pinled output single; mindex local single; tdist local single size=1; debug_motor local boolean; ti local single; tv local; navigate_infrared local; navigate_line local boolean; xc local; yc local; radius local; navigate_avoidboundary local; src output single size=[1 3]; dest output single size=[1 3]; pos_heading output boolean; heading output single; dist output single; data local
  function initialization:
    | function initialization
    | 
    | t1 = single(0); % 0 == no delay time before first state can be entered
    | t2 = single(0); 
    | debug_normal = true; % false == normal mode off
    | debug_motor = false; % false == do not run motor test
    | mindex = single(0); % initialize index for motor test
    | navigate_infrared = false;
    | navigate_line = false;
    | pinled = single(0); % 0 == debug led off
    | tdist = single(40); % 40 == initial distance from rover to target is equal to 40
    | ti = single(1); % 1 == navigate to 1st location
    | tv = single([13 16; 19 16; 13 16; 19 16]); % each row is a target
    | tx = tv(ti,1);
    | ty = tv(ti,2);
    | xc = single(16);
    | yc = single(16);
    | rlimit = single(7);
  function checkrun:
    | function checkrun
    | % check run flag
    | 
    | if sensors.rf == 0
    |     current_task_index = single(2); %not really % stop motor task
    | elseif sensors.rf == 1
    |     current_task_index = single(3); % checkdistance task
    | end
    | 
    | t1 = single(1);
  function stopmotor:
    | function stopmotor
    | % stop motor due to run flag
    | motor_command = single([0 0]);
    | 
    | current_task_index = single(1);
    | if debug_normal == false
    |     t1 = single(10);
    | else
    |     t1 = single(1);
    | end
  function checkdistance:
    | function checkdistance
    | % check the distance of the robot from a target and to the center of the
    | % arena
    | 
    | tdist = calcdistance(tx,ty,sensors.xm,sensors.ym);
    | radius = sqrt((sensors.xm-xc)^2+(sensors.ym-yc)^2);
    | dist = tdist;
    | current_task_index = single(4); % main task
    | t1 = single(1);
  function maintask:
    | function maintask
    | % can use this state to debug and move to a particular state directl
    | 
    | if debug_motor == true
    |     current_task_index = single(7); % motor test state
    | elseif navigate_infrared == true
    |     current_task_index = single(8); % infrared track object state
    | elseif navigate_line == true
    |     current_task_index = single(9); % avoidline state
    | %     elseif navigate_avoidboundary == true
    | %         current_task_index = single(10); % avoid boundary state
    | else
    |     if radius > 7
    |         tx = single(16); ty = single(16);
    |         current_task_index = single(10); % navigate to target x-y
    |     elseif tdist < 1
    |         current_task_index = single(6); % close task
    |     else
    |         current_task_index = single(10); % navigate to target x-y
    |     end
    | end
    |     
    | t1 = single(1);
  function closetask:
    | function closetask
    | % stop motor
    | motor_command = single([0 0]);
    | 
    | % change target when close to current target
    | ti = ti + 1;
    | if (ti > 4)
    |     ti = single(1);  
    | end
    | 
    | tx = tv(ti,1);
    | ty = tv(ti,2);
    | 
    | current_task_index = single(1);
    | if debug_normal == 0
    |     t1 = single(1); % wait before moving onto next location
    | else
    |     t1 = single(1);
    | end
  function test_motor:
    | function test_motor
    | % test motor state
    | 
    | mindex = mindex + 1;
    | % mindex = single(3);
    | if mindex == 1
    |     % move forward
    |     motor_command = single([7 0]);
    |     t1 = single(100);
    | elseif mindex == 2
    |     % move backward
    |     motor_command = single([7 18]);
    |     t1 = single(100);
    | elseif mindex == 3
    |     % spin left
    |     motor_command = single([9 9]);
    |     t1 = single(200);
    | else 
    |     % spin right
    |     motor_command = single([9 27]);
    |     mindex = single(0);
    |     t1 = single(200);
    | end
    | if debug_normal == true
    |     t1 = single(10); % normal mode debug, override t1
    | end
    | current_task_index = single(1);
  function irtrack:
    | function irtrack
    | % check IR distance
    | 
    | persistent found_flag
    | if isempty(found_flag)
    |     found_flag = false;
    | end
    | 
    | t1 = single(1);
    | if sensors.ir >= 150 
    |     % stop moving when close to target
    |     motor_command = single([0 0]);
    | elseif sensors.ir >= 75
    |     if found_flag == false
    |         % turn a litte more until more even with target
    |         motor_command = single([8 9]);
    |         found_flag = true;
    |         t1 = single(150);
    |     else
    |         % move forward until target is reached
    |         motor_command = single([9 0]);
    |     end
    | else
    |     % turn until object is detected
    |     motor_command = single([8 9]);
    | end 
    |         
    | if debug_normal == 1
    |     t1 = single(1); % normal mode debug, override delay time
    | end
    | current_task_index = single(1);
  function avoidline:
    | function avoidline
    | % ls = [front left, front right, back left, back right
    | if sensors.ls(1) == 1 
    |     motor_command = single([7 27]);
    |     t1 = single(200);
    | elseif sensors.ls(2) == 1
    |     motor_command = single([8 9]);
    |     t1 = single(200);
    | else
    |     motor_command = single([9 0]);
    | end
    | 
    | if debug_normal == 1
    |     t1 = single(1); % normal mode debug, override delay time
    | end
    | current_task_index = single(1);
  function testdrewnotsucking:
    | function testdrewnotsucking
    |     
    |     src = single([sensors.xm,sensors.ym,sensors.om]);
    |     dest = single([sensors.xe,sensors.ye,sensors.oe]);
    |     
    |     pos_heading = false;
    |     heading = single(0);
    |     
    |     current_task_index = single(4);
